simulink model "EsquemaCascata"  (R2017a)
settings: Solver=VariableStepAuto  StartTime=0.0  StopTime=50  RelTol=1e-3
settings Model: Creator=julia  LastModifiedBy=julia

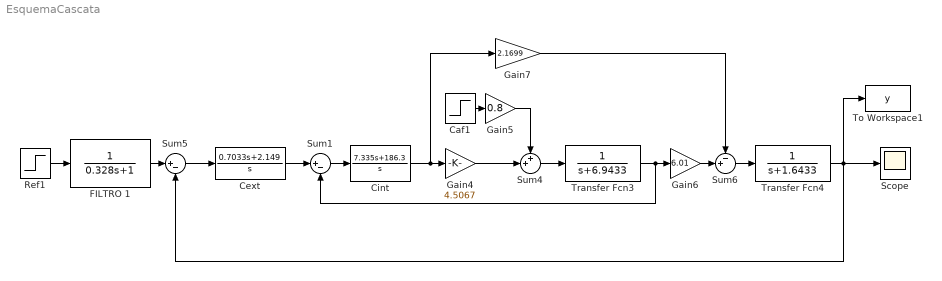
== system EsquemaCascata ==
  Caf1 : Step  Time=20  After=0.05  SampleTime=0
  Cext : TransferFcn  Numerator=[0.7033 2.149]  Denominator=[1 0]
  Cint : TransferFcn  Numerator=[7.335 186.3]  Denominator=[1 0]
  FILTRO 1 : TransferFcn  Numerator=[0 1]  Denominator=[0.328 1]
  Gain4 : Gain  Gain=4.5067
  Gain5 : Gain  Gain=0.8
  Gain6 : Gain  Gain=6.01
  Gain7 : Gain  Gain=2.1699
  Ref1 : Step  Time=0  After=0.1  SampleTime=0
  Scope : Scope
  Sum1 : Sum  Inputs=|+-
  Sum4 : Sum  Inputs=++|
  Sum5 : Sum  Inputs=|+-
  Sum6 : Sum  Inputs=-+|
  To Workspace1 : ToWorkspace  VariableName=y  SaveFormat=Timeseries  SampleTime=-1
  Transfer Fcn3 : TransferFcn  Denominator=[1 6.9433]
  Transfer Fcn4 : TransferFcn  Denominator=[1 1.6433]
  wires:
  Caf1/1 -> Gain5/1
  Gain5/1 -> Sum4/1
  Transfer Fcn4/1 -> Scope/1, To Workspace1/1, Sum5/2
  Sum4/1 -> Transfer Fcn3/1
  Transfer Fcn3/1 -> Sum1/2, Gain6/1
  Ref1/1 -> FILTRO 1/1
  FILTRO 1/1 -> Sum5/1
  Gain4/1 -> Sum4/2
  Sum5/1 -> Cext/1
  Cext/1 -> Sum1/1
  Sum1/1 -> Cint/1
  Cint/1 -> Gain7/1, Gain4/1
  Gain6/1 -> Sum6/2
  Sum6/1 -> Transfer Fcn4/1
  Gain7/1 -> Sum6/1
